simulink model "ThreePhaseHWThyristorSRIND"  (R2014a)
settings: Solver=ode23tb  StartTime=0.0  StopTime=1  RelTol=1e-3
libraries: powerlib x20
settings Model: Creator=ninad gaikawad  LastModifiedBy=ninad gaikawad
settings SolverCC: ZeroCrossAlgorithm=Adaptive
settings DataIOCC: SignalLoggingSaveFormat=ModelDataLogs
settings OptimizationCC: ExpressionDepthLimit=2147483647
settings DebuggingCC: UnderspecifiedInitializationDetection=Classic  FcnCallInpInsideContextMsg=UseLocalSettings  StateNameClashWarn=warning
settings GRTTargetCC: CombineOutputUpdateFcns=off  GRTInterface=on

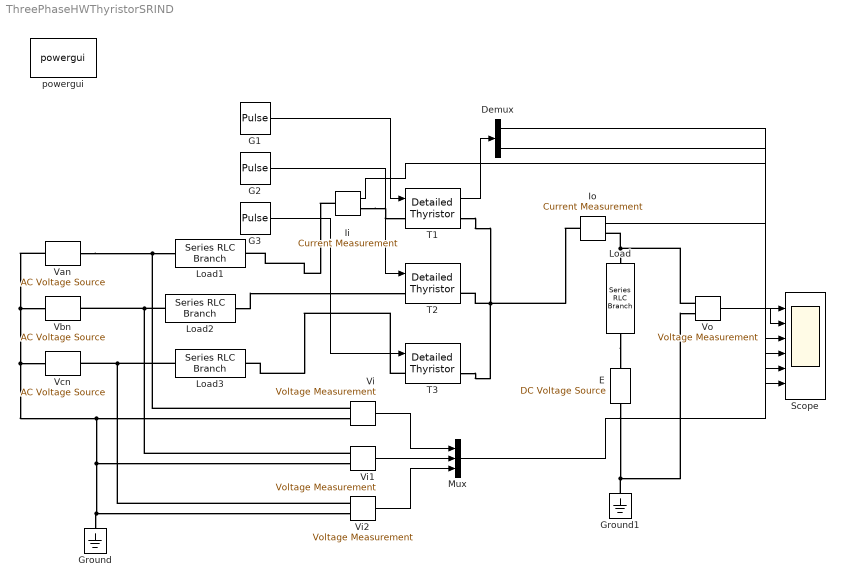
== system ThreePhaseHWThyristorSRIND ==
  Demux : Demux  Outputs=2
  E : powerlib/Electrical Sources/DC Voltage Source  Amplitude=100  Measurements=None
  G1 : DiscretePulseGenerator  PulseType=Time based  Period=20*10^(-3)  PulseWidth=5  PhaseDelay=1/300
  G2 : DiscretePulseGenerator  PulseType=Time based  Period=20*10^(-3)  PulseWidth=5  PhaseDelay=1/300+1/150  VectorParams1D=off
  G3 : DiscretePulseGenerator  PulseType=Time based  Period=20*10^(-3)  PulseWidth=5  PhaseDelay=1/300+2/150
  Ground : powerlib/Elements/Ground  LConnTagsString=a
  Ground1 : powerlib/Elements/Ground  LConnTagsString=a
  Ii : powerlib/Measurements/Current Measurement  PhasorSimulation=off  OutputType=Complex  PSBequivalent=0
  Io : powerlib/Measurements/Current Measurement  PhasorSimulation=off  OutputType=Complex  PSBequivalent=0
  Load : powerlib/Elements/Series RLC Branch  LConnTagsString=__new0  RConnTagsString=__new0  BranchType=RL  Resistance=1  Inductance=0.01  SetiL0=off  InitialCurrent=0  Capacitance=1e-6  Setx0=off  InitialVoltage=0  Measurements=Branch voltage and current
  Load1 : powerlib/Elements/Series RLC Branch  LConnTagsString=__new0  RConnTagsString=__new0  BranchType=L  Resistance=1  Inductance=0.01  SetiL0=off  InitialCurrent=0  Capacitance=1e-6  Setx0=off  InitialVoltage=0  Measurements=Branch voltage and current
  Load2 : powerlib/Elements/Series RLC Branch  LConnTagsString=__new0  RConnTagsString=__new0  BranchType=L  Resistance=1  Inductance=0.01  SetiL0=off  InitialCurrent=0  Capacitance=1e-6  Setx0=off  InitialVoltage=0  Measurements=Branch voltage and current
  Load3 : powerlib/Elements/Series RLC Branch  LConnTagsString=__new0  RConnTagsString=__new0  BranchType=L  Resistance=1  Inductance=0.01  SetiL0=off  InitialCurrent=0  Capacitance=1e-6  Setx0=off  InitialVoltage=0  Measurements=Branch voltage and current
  Mux : Mux  Inputs=3
  Scope : Scope  NumInputPorts=6
      settings: YMin=-5~-5~-5~-5~-5~-5  YMax=5~5~5~5~5~5
  T1 : powerlib/Power Electronics/Detailed Thyristor  Ron=0.001  Lon=1e-3  Vf=0.8  IL=0.1  Tq=100e-6  IC=0  Rs=500  Cs=250e-9  Measurements=on
  T2 : powerlib/Power Electronics/Detailed Thyristor  Ron=0.001  Lon=1e-3  Vf=0.8  IL=0.1  Tq=100e-6  IC=0  Rs=500  Cs=250e-9  Measurements=on
  T3 : powerlib/Power Electronics/Detailed Thyristor  Ron=0.001  Lon=1e-3  Vf=0.8  IL=0.1  Tq=100e-6  IC=0  Rs=500  Cs=250e-9  Measurements=on
  Van : powerlib/Electrical Sources/AC Voltage Source  Amplitude=325  Phase=0  Frequency=50  SampleTime=0  Measurements=None
  Vbn : powerlib/Electrical Sources/AC Voltage Source  Amplitude=325  Phase=-120  Frequency=50  SampleTime=0  Measurements=None
  Vcn : powerlib/Electrical Sources/AC Voltage Source  Amplitude=325  Phase=120  Frequency=50  SampleTime=0  Measurements=None
  Vi : powerlib/Measurements/Voltage Measurement  PhasorSimulation=off  OutputType=Complex  PSBequivalent=0
  Vi1 : powerlib/Measurements/Voltage Measurement  PhasorSimulation=off  OutputType=Complex  PSBequivalent=0
  Vi2 : powerlib/Measurements/Voltage Measurement  PhasorSimulation=off  OutputType=Complex  PSBequivalent=0
  Vo : powerlib/Measurements/Voltage Measurement  PhasorSimulation=off  OutputType=Complex  PSBequivalent=0
  powergui : powerlib/powergui  Priority=1  SimulationMode=Continuous  SolverType=Tustin  SampleTime=50e-6  frequency=60  SPID=off  DisableSnubberDevices=off  DisableRonSwitches=off  DisableVfSwitches=off  SwTol=0  Interpol=off  DisplayEquations=off  Ts=0  methode=off  frequencyindice=50  Pbase=100e6  ErrMax=1e-4  Iterations=50  UnitsV=kV  UnitsW=MW  FunctionMessages=off  echomessages=off  HookPort=off  EnableUseOfTLC=off  x0status=blocks  RestoreLinks=warning  ResistiveCurrentMeasurement=off  Frange=[0:2:500]  Ylog=off  Xlog=on  ShowGrid=off  save=off  variable=ZData  structure=0  ZoomFFT=off  StartTime=0.0  cycles=1  DisplayStyle=1  fundamental=60  FreqAxis=off  MaxFrequency=1000  frequencyindicesteady=1  RmsSteady=1  display=off
  wires:
  Io/1 -> Scope/4
  Demux/2 -> Scope/5
  Demux/1 -> Scope/6
  Vo/1 -> Scope/2
  T1/1 -> Demux/1
  Ii/1 -> Scope/3
  G1/1 -> T1/1
  G2/1 -> T2/1
  G3/1 -> T3/1
  Vi/1 -> Mux/1
  Vi1/1 -> Mux/2
  Vi2/1 -> Mux/3
  Mux/1 -> Scope/1
  connections:
  Load2/RConn1 -- T2/LConn1
  T3/LConn1 -- Load3/RConn1
  T3/RConn1 -- T1/RConn1 -- Io/LConn1 -- T2/RConn1
  Ii/RConn1 -- T1/LConn1
  Ii/LConn1 -- Load1/RConn1
  Vo/LConn1 -- Io/RConn1 -- Load/LConn1
  Vi1/LConn2 -- Vi/LConn2 -- Van/LConn1 -- Vbn/LConn1 -- Vcn/LConn1 -- Vi2/LConn2 -- Ground/LConn1
  Ground1/LConn1 -- E/LConn1 -- Vo/LConn2
  Load/RConn1 -- E/RConn1
  Van/RConn1 -- Vi/LConn1 -- Load1/LConn1
  Load2/LConn1 -- Vi1/LConn1 -- Vbn/RConn1
  Load3/LConn1 -- Vi2/LConn1 -- Vcn/RConn1
